simulink model "processLFP"  (R2012b)
settings: Solver=FixedStepDiscrete  StartTime=0.0  StopTime=10.0  FixedStep=0.001  RelTol=1e-3
settings Model: BufferReuse=off  Creator=gilja  LastModifiedBy=Chethan
settings SolverCC: EnableConcurrentExecution=on  ConcurrentTasks=on
settings DataIOCC: SaveOutput=off  SignalLogging=off  DSMLogging=off  SaveTime=off
settings OptimizationCC: InlineParams=on  InlineInvariantSignals=on  OptimizeBlockIOStorage=off  BufferReuse=off  ExpressionFolding=off  LocalBlockOutputs=off  SimCompilerOptimization=On
settings HardwareCC: ProdIntDivRoundTo=Zero  ProdEndianess=LittleEndian  ProdHWDeviceType=Generic->32-bit x86 compatible
settings ModelReferenceCC: ModelReferenceMinAlgLoopOccurrences=on
settings RTWCC: SystemTargetFile=xpctarget.tlc  TemplateMakefile=xpc_default_tmf  Description=xPC Target  ProcessScript=xpctarget_make_rtw_hook  RTWCompilerOptimization=On
settings CodeAppCC: MaxIdLength=62
settings xpcTargetCC: TargetFcnLib=ansi_tfl_table_tmw.mat  CodeReplacementLibrary=XPC_BLAS  ParMdlRefBuildCompliant=on  ConcurrentExecutionCompliant=on  CombineSignalStateStructs=off  GRTInterface=on  xPCTaskExecutionProfile=on  xPCRL32EventNumber=5000  xPCisDownloadable=off  xPCLoadParamSetFile=off  xPCConcurrentTasks=off  xPCEnableSFAnimation=off

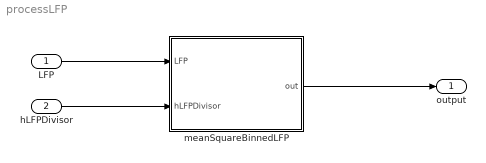
== system processLFP ==
  LFP : Inport  OutDataTypeStr=single
  hLFPDivisor : Inport  Port=2  OutDataTypeStr=double  PortDimensions=1
  meanSquareBinnedLFP : MATLAB Function  TreatAsAtomicUnit=on
  output : Outport  BusOutputAsStruct=on
  wires:
  meanSquareBinnedLFP/1(out) -> output/1
  LFP/1 -> meanSquareBinnedLFP/1(LFP)
  hLFPDivisor/1 -> meanSquareBinnedLFP/2(hLFPDivisor)

== matlab function processLFP/meanSquareBinnedLFP ==
  data: LFP input single size=[1 DecoderConstants.NUM_CHANNELS_PER_ARRAY]; hLFPDivisor input; out output double size=[1 DecoderConstants.NUM_CHANNELS_PER_ARRAY]
function out = procLFP(LFP, hLFPDivisor)
        out = double(LFP.^2) / double(hLFPDivisor);
